simulink model "circuito2branch_working"  (R2018a)
settings: Solver=VariableStepAuto  StartTime=0.0  StopTime=19.5  RelTol=1e-3
undefined symbols (not defined in the file): C1, C2, R0, R1, R2
libraries: powerlib x7
settings Model: Creator=Martin  LastModifiedBy=Martin

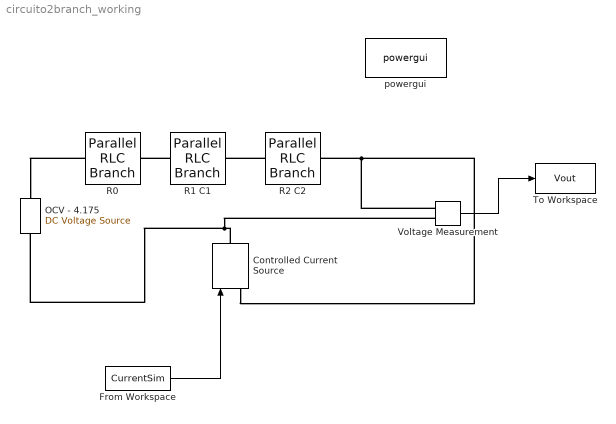
== system circuito2branch_working ==
  Controlled Current Source : powerlib/Electrical Sources/Controlled Current Source  Initialize=on  Source_Type=DC  Amplitude=0  Phase=0  Frequency=0  Measurements=Current
  From Workspace : FromWorkspace  VariableName=CurrentSim  SampleTime=0
  OCV - 4.175 : powerlib/Electrical Sources/DC Voltage Source  Amplitude=4.175  Measurements=None
  R0 : powerlib/Elements/Parallel RLC Branch  LConnTagsString=a  RConnTagsString=__new0  BranchType=R  Resistance=R0  Inductance=0  SetiL0=off  InitialCurrent=0  Capacitance=C1  Setx0=off  InitialVoltage=0  Measurements=Branch voltage
  R1 C1 : powerlib/Elements/Parallel RLC Branch  LConnTagsString=a  RConnTagsString=__new0  BranchType=RC  Resistance=R1  Inductance=0  SetiL0=off  InitialCurrent=0  Capacitance=C1  Setx0=on  InitialVoltage=0  Measurements=Branch voltage
  R2 C2 : powerlib/Elements/Parallel RLC Branch  LConnTagsString=a  RConnTagsString=__new0  BranchType=RC  Resistance=R2  Inductance=0  SetiL0=off  InitialCurrent=0  Capacitance=C2  Setx0=on  InitialVoltage=0  Measurements=Branch voltage
  To Workspace : ToWorkspace  VariableName=Vout  SaveFormat=Timeseries  SampleTime=-1
  Voltage Measurement : powerlib/Measurements/Voltage Measurement  PhasorSimulation=off  OutputType=Complex  PSBequivalent=0
  powergui : powerlib/powergui  Priority=1  SimulationMode=Continuous  SampleTime=50e-6  frequency=60  Iterations=50  frequencyindice=0  Pbase=100e6  ErrMax=1e-4  UnitsV=kV  UnitsW=MW  buscounter=0  FunctionMessages=off  echomessages=off  EnableUseOfTLC=off  CurrentSourceSwitches=off  DisableSnubberDevices=off  DisableRonSwitches=off  DisableVfSwitches=off  DisplayEquations=off  SolverType=Tustin/Backward Euler (TBE)  Interpol=off  ExternalGateDelay=off  methode=off  Ts=100  x0status=blocks  SPID=on  SwTol=0  HookPort=off  RestoreLinks=warning  ResistiveCurrentMeasurement=off  Frange=[0:2:500]  Ylog=off  Xlog=on  ShowGrid=off  save=off  variable=ZData  structure=0  ZoomFFT=off  StartTime=0.0  cycles=1  DisplayStyle=1  fundamental=60  FreqAxis=off  MaxFrequency=1000  frequencyindicesteady=1  RmsSteady=1  display=off
  wires:
  Voltage Measurement/1 -> To Workspace/1
  From Workspace/1 -> Controlled Current Source/1
  connections:
  R2 C2/LConn1 -- R1 C1/RConn1
  Controlled Current Source/RConn1 -- Voltage Measurement/LConn2 -- OCV - 4.175/LConn1
  R0/LConn1 -- OCV - 4.175/RConn1
  R1 C1/LConn1 -- R0/RConn1
  Controlled Current Source/LConn1 -- Voltage Measurement/LConn1 -- R2 C2/RConn1
